simulink model "manipulator_CBF_cvxpy"  (R2024a)
settings: Solver=FixedStepAuto  StartTime=0.0  StopTime=Tf  FixedStep=Ts  RelTol=1e-3
undefined symbols (not defined in the file): gamma, init_q, InitPos, u_des
libraries: robotmaniplib x1
settings Model: Creator=bumyong  LastModifiedBy=bumyong

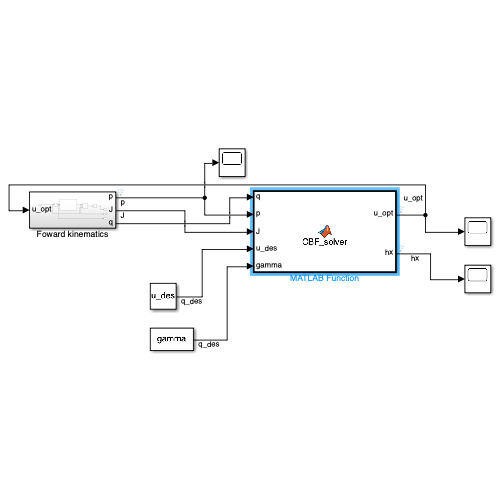
[thumbnail: Simulink's stored preview of the top-level diagram]
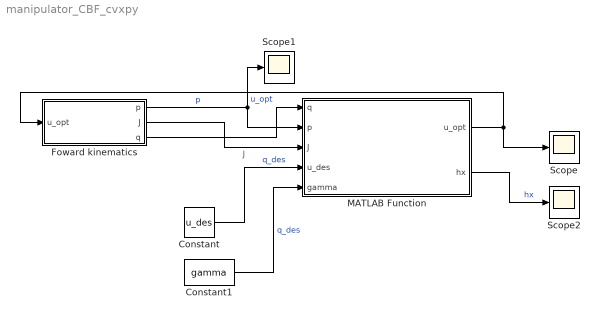
== system manipulator_CBF_cvxpy ==
  Constant : Constant  Value=u_des
  Constant1 : Constant  Value=gamma
  Foward kinematics : Subsystem
  MATLAB Function : MATLAB Function  TreatAsAtomicUnit=on
  Scope : Scope
  Scope1 : Scope
  Scope2 : Scope
  wires:
  Constant/1 -> MATLAB Function/4(u_des)  "q_des"
  Constant1/1 -> MATLAB Function/5(gamma)  "q_des"
  Foward kinematics/1(p) -> MATLAB Function/2(p), Scope1/1  "p"
  Foward kinematics/2(J) -> MATLAB Function/3(J)  "J"
  Foward kinematics/3(q) -> MATLAB Function/1(q)
  MATLAB Function/1(u_opt) -> Scope/1, Foward kinematics/1(u_opt)  "u_opt"
  MATLAB Function/2(hx) -> Scope2/1  "hx"

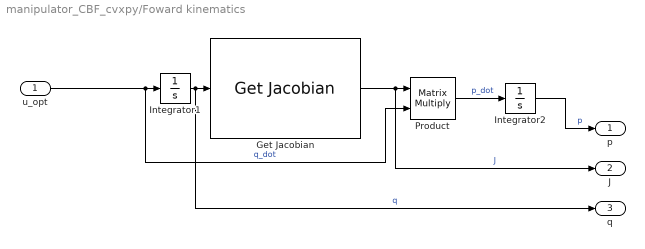
== system manipulator_CBF_cvxpy/Foward kinematics ==
  u_opt : Inport
  Get Jacobian : robotmaniplib/Get Jacobian  RigidBodyTree=robot  EndEffector=link7  SimulateUsing=Interpreted execution
  Integrator1 : Integrator  InitialCondition=init_q
  Integrator2 : Integrator  InitialCondition=[0;0;0;InitPos]
  Product : Product  Multiplication=Matrix(*)
  p : Outport
  J : Outport  Port=2
  q : Outport  Port=3
  wires:
  Integrator1/1 -> q/1, Get Jacobian/1  "q"
  Product/1 -> Integrator2/1  "p_dot"
  u_opt/1 -> Product/2, Integrator1/1  "q_dot"
  Get Jacobian/1 -> J/1, Product/1  "J"
  Integrator2/1 -> p/1  "p"

== matlab function manipulator_CBF_cvxpy/MATLAB Function ==
  data: q input; u_opt output; p input; J input; u_des input; gamma input; hx output
function [u_opt, hx]  = CBF_solver(q, p, J, u_des, gamma)

    u_opt = double([0 0 0 0 0 0]');
    hx = double(0);

    p_obs = [0 0.4 1]'; % Position of the obstacle
    R = 0.1; % Radious of the obstacle
    R_w = 0.1; % Radious of the wrist of robot

    coder.extrinsic('py.manipulator_CBF_cvxpy.manipulator_cbf');


    result = py.manipulator_CBF_cvxpy.manipulator_cbf(q, p(4:6), J, u_des, gamma);
    hx = norm(p(4:6) - p_obs)^2 - (R + R_w)^2;

    u_opt = double(result)';
end
